simulink library "mlepLibrary"  (R2021a)
settings: Solver=ode45  StartTime=0.0  StopTime=10.0  RelTol=1e-3
undefined symbols (not defined in the file or in its folder): mlepEnergyPlusSimulation_clbk, vector2Bus_clbk
settings Model: Creator=willyg  LastModifiedBy=migue
settings SolverCC: AlgebraicLoopSolver=TrustRegion
settings DataIOCC: LimitDataPoints=on  SaveFormat=Array  SignalLoggingSaveFormat=ModelDataLogs
settings OptimizationCC: BlockReduction=off  BooleanDataType=off  LifeSpan=inf
settings DebuggingCC: SaveWithParameterizedLinksMsg=none  UnderspecifiedInitializationDetection=Classic  MergeDetectMultiDrivingBlocksExec=none  SignalResolutionControl=TryResolveAllWithWarning  MultiTaskDSMMsg=warning  MultiTaskCondExecSysMsg=none  SFUnexpectedBacktrackingDiag=warning  SFNoUnconditionalDefaultTransitionDiag=warning  SFExecutionAtInitializationDiag=none  SFMachineParentedDataDiag=warning  ArithmeticOperatorsInVariantConditions=warning
settings HardwareCC: ProdBitPerPointer=32  ProdBitPerSizeT=32  ProdBitPerPtrDiffT=32  ProdLargestAtomicFloat=None  ProdIntDivRoundTo=Undefined  ProdEndianess=Unspecified  ProdWordSize=32  ProdHWDeviceType=32-bit Generic  TargetUnknown=on
settings ModelReferenceCC: PropagateSignalLabelsOutOfModel=off
settings SFSimCC: SimUseLocalCustomCode=off  CustomCodeUndefinedFunction=UseInterfaceOnly
settings RTWCC: RTWUseLocalCustomCode=off
settings CodeAppCC: StateflowObjectComments=on
settings GRTTargetCC: TargetLangStandard=C89/C90 (ANSI)
settings ConfigComp: CovMetricSettings=dw  CovSaveCumulativeToWorkspaceVar=on  CovSaveSingleToWorkspaceVar=on  CovExternalEMLEnable=off

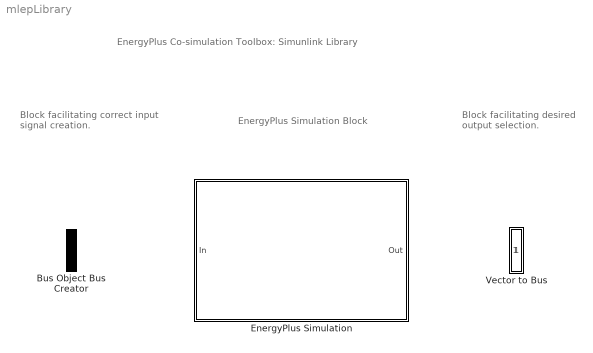
== system mlepLibrary ==
  note: EnergyPlus Simulation Block
  note: EnergyPlus Co-simulation Toolbox: Simunlink Library
  note: Block facilitating correct
      | input signal creation.
  note: Block facilitating desired
      | output selection.
  Bus Object Bus Creator : BusCreator  Priority=2  Inputs=1  mask(Bus Object Bus Creator){busType=Select a Bus object...}
      mask prompts: busType "Bus Type"
      mask help:
      | Provides users the cabability to painlessly, instantly customize bus creators of output data type 'Bus:' by selecting the bus object type from a drop down menu dynamically populated by bus objects in the workspace.
      |
      | After pressing the "Create named signals" button signal lines into the creator are populated and named with the elements in the chosen bus saving the user from having to recall and fill out signal line names.
      settings: AttributesFormatString=%<OutDataTypeStr>  CopyFcn=busObjectBusCreator_clbk(gcb,'CopyFcn');
      mask TypeOptions busType: Select a Bus object... | Bus: epInbus | Bus: epInbusCopy | Bus: epOutbus
      mask Callback busType: busObjectBusCreator_clbk(gcb,'popup');
      mask DialogControl applyMOCBSelection Prompt: Create named signals
      mask DialogControl applyMOCBSelection Callback: busObjectBusCreator_clbk(gcb,'button');
  EnergyPlus Simulation : Subsystem  Priority=1  InitFcn=mlepEnergyPlusSimulation_clbk(gcb,'InitFcn');  mask(EP communication block){idfFile=, epwFile=, inputBusName=epInbus, outputBusName=epOutbus, useDataDictionary=off, dataDictionaryName=EnergyPlusSimulation.sldd}
      mask prompts: idfFile "Specify IDF file:"; epwFile "Specify EPW file:"; inputBusName "Input bus name:"; outputBusName "Output bus name:"; useDataDictionary "Store Bus objects in Data dictionary?"; dataDictionaryName "Data Dictionary:"
      mask help: Run EnergyPlus process, prepare simulation of the IDF file, establish communication and co-simulate using Matlab inputs and EnergyPlus outputs.
      mask init:
      | %mlepEnergyPlusSimulation_clbk(gcb, 'maskInit');
      settings: OpenFcn=mlepEnergyPlusSimulation_clbk(gcb,'OpenFcn');
      mask Help: web([fileparts(which('setupMlep.m')) '\doc\' 'GettingStarted.html'])
      mask TypeOptions idfFile: mlep System Object/idfFile
      mask TypeOptions epwFile: mlep System Object/epwFile
      mask TypeOptions inputBusName: mlep System Object/inputBusName
      mask TypeOptions outputBusName: mlep System Object/outputBusName
      mask TypeOptions useDataDictionary: mlep System Object/useDataDictionary
      mask TypeOptions dataDictionaryName: mlep System Object/dataDictionaryName
      mask DialogControl Container4 Prompt: Simulation
      mask DialogControl Control2 Prompt: Browse
      mask DialogControl Control2 Callback: mlepEnergyPlusSimulation_clbk(gcb,'browseButton','IDF');
      mask DialogControl Control3 Prompt: Browse
      mask DialogControl Control3 Callback: mlepEnergyPlusSimulation_clbk(gcb,'browseButton','EPW');
      mask DialogControl Container16 Prompt: Bus
      mask DialogControl Control4 Prompt: Generate Bus Objects
      mask DialogControl Control4 Callback: mlepEnergyPlusSimulation_clbk(gcb,'generateBus');
      mask Display: block_icon('mlep System Object');
  Vector to Bus : Subsystem  InitFcn=vector2Bus_clbk(gcb,'InitFcn');  mask{busType=Select a Bus object...}
      mask prompts: busType "Bus Type"
      mask init:
      | vector2Bus_clbk(gcb,'maskInit');
      settings: AttributesFormatString=%<busType>  CopyFcn=vector2Bus_clbk(gcb,'CopyFcn');
      mask TypeOptions busType: Select a Bus object... | Bus: epInbusCopy | Bus: epOutbus
      mask Callback busType: vector2Bus_clbk(gcb,'popup');
      mask Display:
      | % Black background
      | % patch([0 1 1 0 0],[0 0 1 1 0],[0 0 0]);
      | 
      | % Text
      | color white
      | fprintf('V\n2\nB')

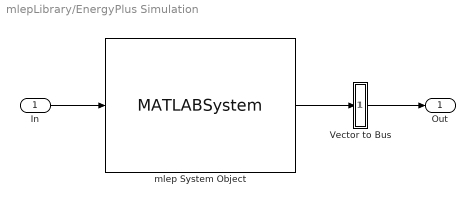
== system mlepLibrary/EnergyPlus Simulation ==
  In : Inport  OutDataTypeStr=Bus: epInbus
  Vector to Bus : Subsystem  InitFcn=vector2Bus_clbk(gcb,'InitFcn');  mask{busType=Select a Bus object...}
      mask prompts: busType "Bus Type"
      mask init:
      | vector2Bus_clbk(gcb,'maskInit');
      settings: AttributesFormatString=%<busType>
      mask TypeOptions busType: Select a Bus object... | Bus: epInbusCopy | Bus: epOutbus
      mask Callback busType: vector2Bus_clbk(gcb,'popup');
      mask Display:
      | % Black background
      | % patch([0 1 1 0 0],[0 0 1 1 0],[0 0 0]);
      | 
      | % Text
      | color white
      | fprintf('V\n2\nB')
  mlep System Object : MATLABSystem  Priority=1  System=mlep  inputBusName=epInbus  outputBusName=epOutbus  useDataDictionary=off  dataDictionaryName=EnergyPlusSimulation.sldd
      mask Type: mlep
      mask Display:
      | image('mlepIcon.jpg');
      | port_label('input',1,'epInbus');
      | port_label('output',1,'epOutbus');
  Out : Outport  OutDataTypeStr=Bus: epOutbus
  wires:
  In/1 -> mlep System Object/1
  mlep System Object/1 -> Vector to Bus/1(In1)
  Vector to Bus/1(Out1) -> Out/1

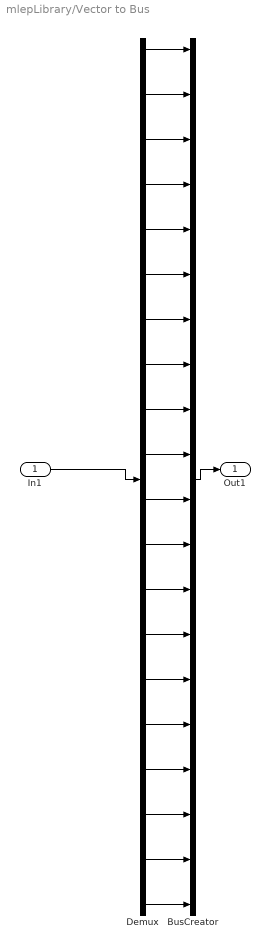
== system mlepLibrary/Vector to Bus ==
  In1 : Inport
  BusCreator : BusCreator  Inputs=20
  Demux : Demux  Outputs=20
  Out1 : Outport
  wires:
  In1/1 -> Demux/1
  BusCreator/1 -> Out1/1
  Demux/1 -> BusCreator/1
  Demux/2 -> BusCreator/2
  Demux/3 -> BusCreator/3
  Demux/4 -> BusCreator/4
  Demux/5 -> BusCreator/5
  Demux/6 -> BusCreator/6
  Demux/7 -> BusCreator/7
  Demux/8 -> BusCreator/8
  Demux/9 -> BusCreator/9
  Demux/10 -> BusCreator/10
  Demux/11 -> BusCreator/11
  Demux/12 -> BusCreator/12
  Demux/13 -> BusCreator/13
  Demux/14 -> BusCreator/14
  Demux/15 -> BusCreator/15
  Demux/16 -> BusCreator/16
  Demux/17 -> BusCreator/17
  Demux/18 -> BusCreator/18
  Demux/19 -> BusCreator/19
  Demux/20 -> BusCreator/20

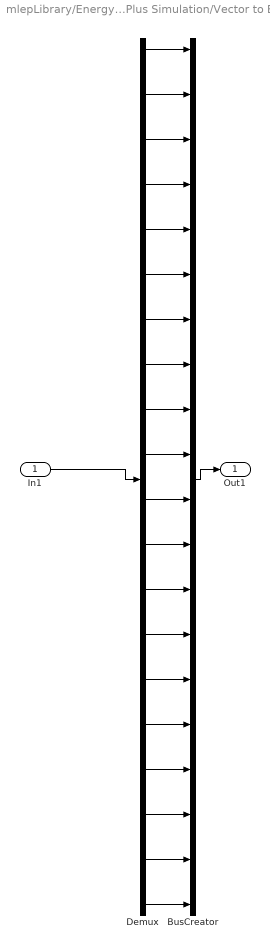
== system mlepLibrary/EnergyPlus Simulation/Vector to Bus ==
  In1 : Inport
  BusCreator : BusCreator  Inputs=20
  Demux : Demux  Outputs=20
  Out1 : Outport
  wires:
  In1/1 -> Demux/1
  BusCreator/1 -> Out1/1
  Demux/1 -> BusCreator/1
  Demux/2 -> BusCreator/2
  Demux/3 -> BusCreator/3
  Demux/4 -> BusCreator/4
  Demux/5 -> BusCreator/5
  Demux/6 -> BusCreator/6
  Demux/7 -> BusCreator/7
  Demux/8 -> BusCreator/8
  Demux/9 -> BusCreator/9
  Demux/10 -> BusCreator/10
  Demux/11 -> BusCreator/11
  Demux/12 -> BusCreator/12
  Demux/13 -> BusCreator/13
  Demux/14 -> BusCreator/14
  Demux/15 -> BusCreator/15
  Demux/16 -> BusCreator/16
  Demux/17 -> BusCreator/17
  Demux/18 -> BusCreator/18
  Demux/19 -> BusCreator/19
  Demux/20 -> BusCreator/20
